simulink model "sin_cos"  (R2018b)
settings: Solver=FixedStepAuto  StartTime=0.0  StopTime=10.0  FixedStep=0.01  RelTol=1e-3
settings Model: Creator=Ismael  LastModifiedBy=Ismael

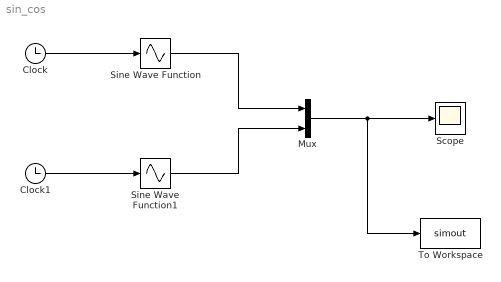
== system sin_cos ==
  Clock : Clock
  Clock1 : Clock
  Mux : Mux  Inputs=2
  Scope : Scope
  Sine Wave Function : Sin  TimeSource=Use external signal  SampleTime=0
  Sine Wave Function1 : Sin  TimeSource=Use external signal  Phase=pi/2  SampleTime=0
  To Workspace : ToWorkspace  VariableName=simout  SampleTime=-1
  wires:
  Clock/1 -> Sine Wave Function/1
  Sine Wave Function1/1 -> Mux/2
  Sine Wave Function/1 -> Mux/1
  Mux/1 -> To Workspace/1, Scope/1
  Clock1/1 -> Sine Wave Function1/1
